simulink model "Drone_model"  (R2021a)
settings: Solver=VariableStepAuto  StartTime=0.0  StopTime=10.0  RelTol=1e-3
settings Model: Creator=David  LastModifiedBy=David

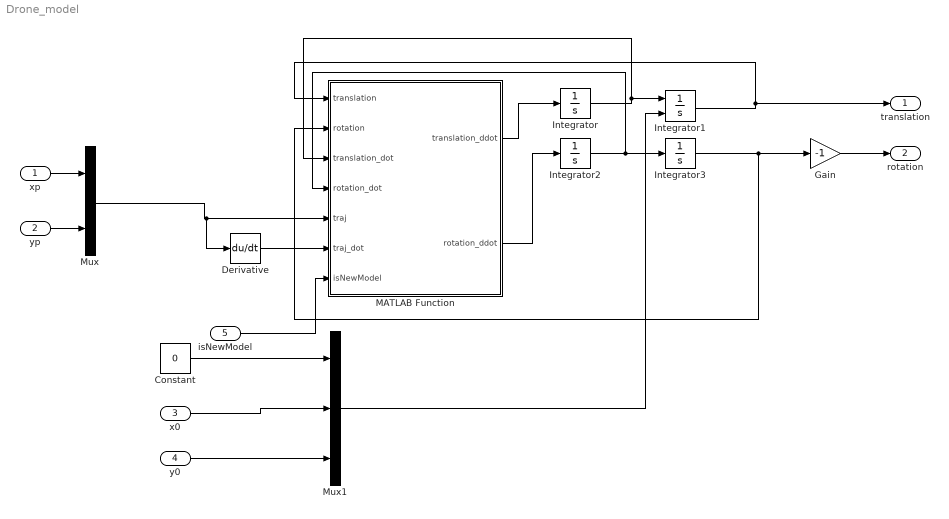
== system Drone_model ==
  xp : Inport
  yp : Inport  Port=2
  x0 : Inport  Port=3
  y0 : Inport  Port=4
  isNewModel : Inport  Port=5  OutDataTypeStr=boolean
  Constant : Constant  Value=0
  Derivative : Derivative
  Gain : Gain  Gain=-1
  Integrator : Integrator  InitialCondition=[0,0,0]
  Integrator1 : Integrator  InitialConditionSource=external  InitialCondition=[1,1,1]
  Integrator2 : Integrator  InitialCondition=[0,0,0]
  Integrator3 : Integrator  InitialCondition=[0,0,0]
  MATLAB Function : MATLAB Function  TreatAsAtomicUnit=on
  Mux : Mux  Inputs=2
  Mux1 : Mux  Inputs=3
  translation : Outport
  rotation : Outport  Port=2
  wires:
  MATLAB Function/2(rotation_ddot) -> Integrator2/1
  MATLAB Function/1(translation_ddot) -> Integrator/1
  Integrator3/1 -> Gain/1, MATLAB Function/2(rotation)
  Integrator/1 -> Integrator1/1, MATLAB Function/3(translation_dot)
  Integrator1/1 -> translation/1, MATLAB Function/1(translation)
  Integrator2/1 -> MATLAB Function/4(rotation_dot), Integrator3/1
  xp/1 -> Mux/1
  yp/1 -> Mux/2
  Mux/1 -> Derivative/1, MATLAB Function/5(traj)
  Mux1/1 -> Integrator1/2
  Constant/1 -> Mux1/1
  y0/1 -> Mux1/3
  x0/1 -> Mux1/2
  Gain/1 -> rotation/1
  isNewModel/1 -> MATLAB Function/7(isNewModel)
  Derivative/1 -> MATLAB Function/6(traj_dot)

== matlab function Drone_model/MATLAB Function ==
  data: translation input; translation_ddot output; rotation input; rotation_ddot output; translation_dot input; rotation_dot input; traj input; traj_dot input; isNewModel input
function [translation_ddot,rotation_ddot] = fcn(translation,rotation,translation_dot,rotation_dot,traj,traj_dot,isNewModel)
    drone_obj=Drone(isNewModel);
    [translation_ddot,rotation_ddot]=drone_obj.Compute_state(translation,rotation,...
        translation_dot,rotation_dot,traj,traj_dot);
